simulink model "AdaptedGliderModel"  (R2019b)
settings: Solver=VariableStepAuto  StartTime=0.0  StopTime=10.0  RelTol=1e-3
undefined symbols (not defined in the file or in its folder): MDL
libraries: simulink x4, Driver_Glider_Library x2
settings Model: Creator=eduar  LastModifiedBy=eduar

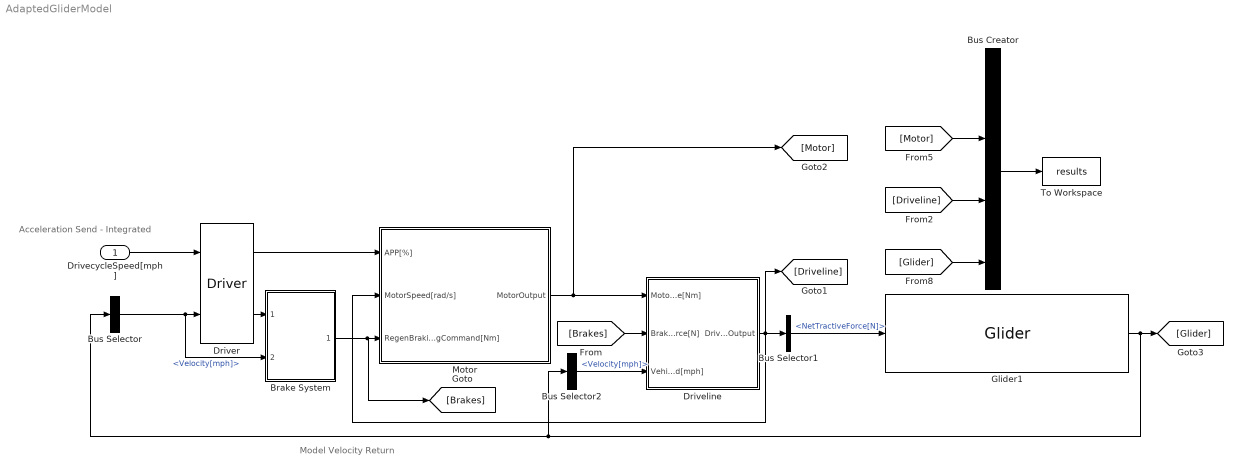
== system AdaptedGliderModel ==
  note: Model Velocity Return
  note: Acceleration Send - Integrated
  DrivecycleSpeed[mph] : Inport
  Brake System : Subsystem
      mask Display: image('brakes.jpg');
  Bus Creator : BusCreator  Inputs=4
  Bus Selector : BusSelector  OutputSignals=Velocity[mph]
  Bus Selector1 : BusSelector  OutputSignals=NetTractiveForce[N]
  Bus Selector2 : BusSelector  OutputSignals=Velocity[mph]
  Driveline : Subsystem
      mask Display: image('driveline.jpg');
  Driver : Driver_Glider_Library/Driver  SystemSampleTime=-1  Latency=0  AutoFrameSizeCalculation=off
  Glider1 : Driver_Glider_Library/Glider  SystemSampleTime=-1  Latency=0  AutoFrameSizeCalculation=off
      link override AerodynamicDrag[N]: Gain=0
      link override Force2Acceleration: Gain=1/388
      link override GradeForce[N]: Value=0
      link override RollingResistance[N]: Value=388*9.8*rollingResistCoeff
  Motor : Subsystem
      mask Display: image('motor.jpg');
  To Workspace : ToWorkspace  VariableName=results  SaveFormat=Timeseries  SampleTime=-1
  wires:
  Driver/1 -> Motor/1(APP[%])
  Bus Selector1/1 -> Glider1/1  "<NetTractiveForce[N]>"
  Bus Selector/1 -> Brake System/2(VehicleSpeed[mph]), Driver/2  "<Velocity[mph]>"
  Driver/2 -> Brake System/1(BPP[%])
  [Motor] -> Bus Creator/2
  DrivecycleSpeed[mph]/1 -> Driver/1
  Bus Creator/1 -> To Workspace/1
  Glider1/1 -> [Glider], Bus Selector/1, Bus Selector2/1
  [Driveline] -> Bus Creator/3
  Driveline/1(DrivelineOutput) -> Bus Selector1/1, Motor/2(MotorSpeed[rad/s]), [Driveline]
  Motor/1(MotorOutput) -> [Motor], Driveline/1(MotorTorque[Nm])
  [Glider] -> Bus Creator/4
  Brake System/1(BrakeOutput) -> [Brakes], Motor/3(RegenBrakingCommand[Nm])
  Bus Selector2/1 -> Driveline/3(VehicleSpeed[mph])  "<Velocity[mph]>"
  [Brakes] -> Driveline/2(BrakeForce[N])

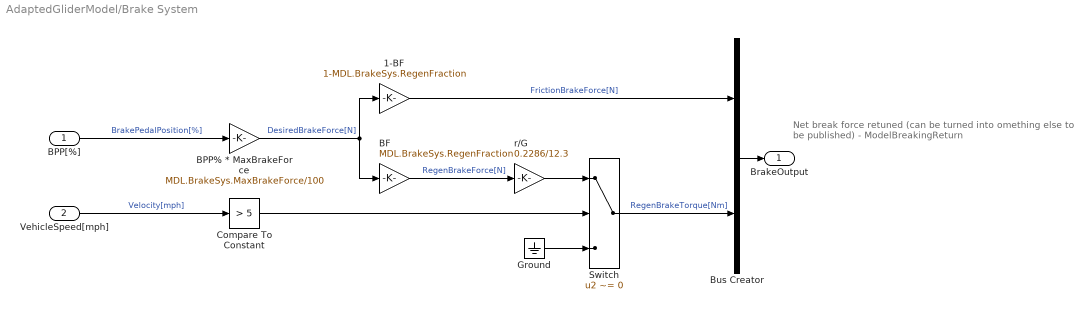
== system AdaptedGliderModel/Brake System ==
  note: Net break force retuned (can be turned into omething else
      | to be published) - ModelBreakingReturn
  BPP[%] : Inport
  VehicleSpeed[mph] : Inport  Port=2
  1-BF : Gain  Gain=1-MDL.BrakeSys.RegenFraction
  BF : Gain  Gain=MDL.BrakeSys.RegenFraction
  BPP% * MaxBrakeForce : Gain  Gain=MDL.BrakeSys.MaxBrakeForce/100
  Bus Creator : BusCreator  Inputs=2
  Compare To Constant : simulink/Logic and Bit Operations/Compare To Constant  relop=>  const=5  OutDataTypeStr=boolean
  Ground : Ground
  Switch : Switch  Criteria=u2 ~= 0
  r/G : Gain  Gain=0.2286/12.3
  BrakeOutput : Outport  VectorParamsAs1DForOutWhenUnconnected=off
  wires:
  Bus Creator/1 -> BrakeOutput/1
  BPP[%]/1 -> BPP% * MaxBrakeForce/1  "BrakePedalPosition[%]"
  BPP% * MaxBrakeForce/1 -> BF/1, 1-BF/1  "DesiredBrakeForce[N]"
  BF/1 -> r/G/1  "RegenBrakeForce[N]"
  1-BF/1 -> Bus Creator/1  "FrictionBrakeForce[N]"
  r/G/1 -> Switch/1
  VehicleSpeed[mph]/1 -> Compare To Constant/1  "Velocity[mph]"
  Ground/1 -> Switch/3
  Switch/1 -> Bus Creator/2  "RegenBrakeTorque[Nm]"
  Compare To Constant/1 -> Switch/2

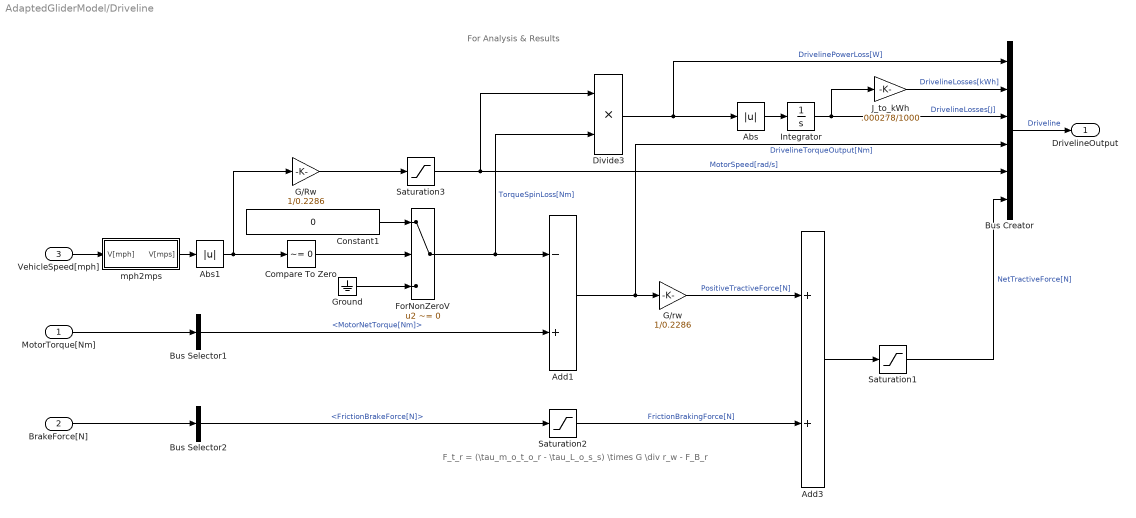
== system AdaptedGliderModel/Driveline ==
  note: For Analysis & Results
  note: F_t_r = (\tau_m_o_t_o_r - \tau_L_o_s_s) \times G \div r_w - F_B_r
  MotorTorque[Nm] : Inport
  BrakeForce[N] : Inport  Port=2
  VehicleSpeed[mph] : Inport  Port=3
  Abs : Abs  ZeroCross=off
  Abs1 : Abs  ZeroCross=off
  Add1 : Sum  Inputs=-+
  Add3 : Sum
  Bus Creator : BusCreator  Inputs=6
  Bus Selector1 : BusSelector  OutputSignals=MotorNetTorque[Nm]
  Bus Selector2 : BusSelector  OutputSignals=FrictionBrakeForce[N]
  Compare To Zero : simulink/Logic and Bit Operations/Compare To Zero  relop=~=  OutDataTypeStr=boolean
  Constant1 : Constant  Value=0
  Divide3 : Product  Inputs=**
  ForNonZeroV : Switch  Criteria=u2 ~= 0  ZeroCross=off
  G/Rw : Gain  Gain=1/0.2286
  G/rw : Gain  Gain=1/0.2286
  Ground : Ground
  Integrator : Integrator  ZeroCross=off
  J_to_kWh : Gain  Gain=.000278/1000
  Saturation1 : Saturate  UpperLimit=5000  LowerLimit=-10000  ZeroCross=off
  Saturation2 : Saturate  UpperLimit=0  LowerLimit=-10000  ZeroCross=off
  Saturation3 : Saturate  UpperLimit=inf  LowerLimit=0.00001  ZeroCross=off
  mph2mps : Subsystem
  DrivelineOutput : Outport  VectorParamsAs1DForOutWhenUnconnected=off
  wires:
  G/rw/1 -> Add3/1  "PositiveTractiveForce[N]"
  Add3/1 -> Saturation1/1
  Abs/1 -> Integrator/1
  BrakeForce[N]/1 -> Bus Selector2/1
  Saturation2/1 -> Add3/2  "FrictionBrakingForce[N]"
  MotorTorque[Nm]/1 -> Bus Selector1/1
  G/Rw/1 -> Saturation3/1
  VehicleSpeed[mph]/1 -> mph2mps/1(V[mph])
  ForNonZeroV/1 -> Divide3/2, Add1/1  "TorqueSpinLoss[Nm]"
  Add1/1 -> Bus Creator/4, G/rw/1  "DrivelineTorqueOutput[Nm]"
  Saturation3/1 -> Divide3/1, Bus Creator/5  "MotorSpeed[rad/s]"
  Divide3/1 -> Bus Creator/1, Abs/1  "DrivelinePowerLoss[W]"
  Saturation1/1 -> Bus Creator/6  "NetTractiveForce[N]"
  Abs1/1 -> Compare To Zero/1, G/Rw/1
  Bus Selector2/1 -> Saturation2/1  "<FrictionBrakeForce[N]>"
  J_to_kWh/1 -> Bus Creator/2  "DrivelineLosses[kWh]"
  Ground/1 -> ForNonZeroV/3
  Constant1/1 -> ForNonZeroV/1
  Bus Creator/1 -> DrivelineOutput/1  "Driveline"
  Integrator/1 -> J_to_kWh/1, Bus Creator/3  "DrivelineLosses[J]"
  Bus Selector1/1 -> Add1/2  "<MotorNetTorque[Nm]>"
  Compare To Zero/1 -> ForNonZeroV/2
  mph2mps/1(V[mps]) -> Abs1/1

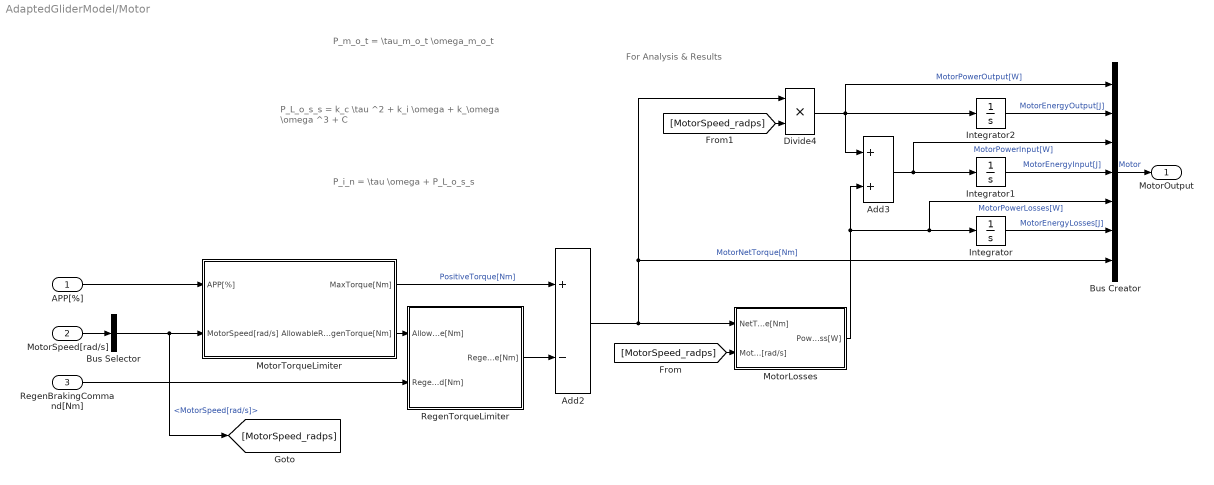
== system AdaptedGliderModel/Motor ==
  note: P_i_n = \tau \omega + P_L_o_s_s
  note: For Analysis & Results
  note: P_L_o_s_s = k_c \tau ^2 + k_i \omega + k_\omega \omega ^3 + C
  note: P_m_o_t = \tau_m_o_t \omega_m_o_t
  APP[%] : Inport
  MotorSpeed[rad/s] : Inport  Port=2
  RegenBrakingCommand[Nm] : Inport  Port=3
  Add2 : Sum  Inputs=+-
  Add3 : Sum
  Bus Creator : BusCreator  Inputs=7
  Bus Selector : BusSelector  OutputSignals=MotorSpeed[rad/s]
  Divide4 : Product  Inputs=**
  Integrator : Integrator  ZeroCross=off
  Integrator1 : Integrator  ZeroCross=off
  Integrator2 : Integrator  ZeroCross=off
  MotorLosses : Subsystem
  MotorTorqueLimiter : Subsystem
  RegenTorqueLimiter : Subsystem
  MotorOutput : Outport  VectorParamsAs1DForOutWhenUnconnected=off
  wires:
  Add3/1 -> Bus Creator/3, Integrator1/1  "MotorPowerInput[W]"
  Divide4/1 -> Bus Creator/1, Add3/1, Integrator2/1  "MotorPowerOutput[W]"
  [MotorSpeed_radps] -> Divide4/2
  Integrator1/1 -> Bus Creator/4  "MotorEnergyInput[J]"
  Integrator2/1 -> Bus Creator/2  "MotorEnergyOutput[J]"
  Add2/1 -> MotorLosses/1(NetTorque[Nm]), Divide4/1, Bus Creator/7  "MotorNetTorque[Nm]"
  MotorTorqueLimiter/1(MaxTorque[Nm]) -> Add2/1  "PositiveTorque[Nm]"
  APP[%]/1 -> MotorTorqueLimiter/1(APP[%])
  MotorLosses/1(PowerLoss[W]) -> Bus Creator/5, Integrator/1, Add3/2  "MotorPowerLosses[W]"
  RegenBrakingCommand[Nm]/1 -> RegenTorqueLimiter/2(RegenBrakeCommand[Nm])
  MotorTorqueLimiter/2(AllowableRegenTorque[Nm]) -> RegenTorqueLimiter/1(AllowableRegenTorque[Nm])
  RegenTorqueLimiter/1(RegenTorque[Nm]) -> Add2/2
  [MotorSpeed_radps] -> MotorLosses/2(MotorSpeed[rad/s])
  Bus Creator/1 -> MotorOutput/1  "Motor"
  Integrator/1 -> Bus Creator/6  "MotorEnergyLosses[J]"
  MotorSpeed[rad/s]/1 -> Bus Selector/1
  Bus Selector/1 -> MotorTorqueLimiter/2(MotorSpeed[rad/s]), [MotorSpeed_radps]  "<MotorSpeed[rad/s]>"

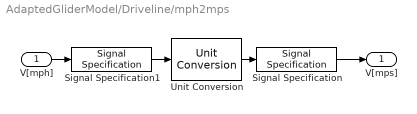
== system AdaptedGliderModel/Driveline/mph2mps ==
  V[mph] : Inport
  Signal Specification : SignalSpecification  Unit=m/s
  Signal Specification1 : SignalSpecification  Unit=mile/hr
  Unit Conversion : UnitConversion
  V[mps] : Outport  VectorParamsAs1DForOutWhenUnconnected=off
  wires:
  V[mph]/1 -> Signal Specification1/1
  Unit Conversion/1 -> Signal Specification/1
  Signal Specification1/1 -> Unit Conversion/1
  Signal Specification/1 -> V[mps]/1

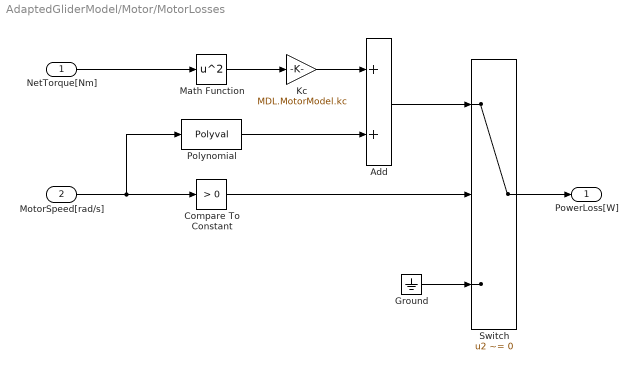
== system AdaptedGliderModel/Motor/MotorLosses ==
  NetTorque[Nm] : Inport
  MotorSpeed[rad/s] : Inport  Port=2
  Add : Sum
  Compare To Constant : simulink/Logic and Bit Operations/Compare To Constant  relop=>  const=0  OutDataTypeStr=boolean
  Ground : Ground
  Kc : Gain  Gain=MDL.MotorModel.kc
  Math Function : Math  Operator=square  SaturateOnIntegerOverflow=on
  Polynomial : Polyval  Coefs=[MDL.MotorModel.kw , 0 ,MDL.MotorModel.ki, MDL.MotorModel.C]
  Switch : Switch  Criteria=u2 ~= 0  ZeroCross=off
  PowerLoss[W] : Outport  VectorParamsAs1DForOutWhenUnconnected=off
  wires:
  NetTorque[Nm]/1 -> Math Function/1
  Math Function/1 -> Kc/1
  Kc/1 -> Add/1
  MotorSpeed[rad/s]/1 -> Polynomial/1, Compare To Constant/1
  Ground/1 -> Switch/3
  Switch/1 -> PowerLoss[W]/1
  Polynomial/1 -> Add/2
  Add/1 -> Switch/1
  Compare To Constant/1 -> Switch/2

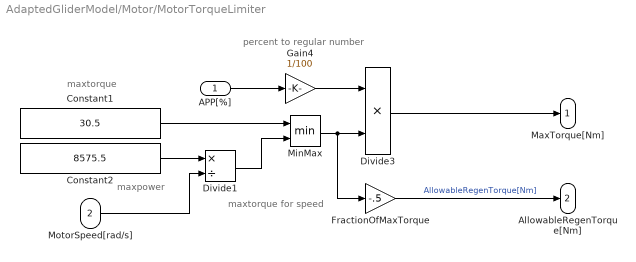
== system AdaptedGliderModel/Motor/MotorTorqueLimiter ==
  note: percent to regular number
  note: maxtorque for speed
  note: maxtorque
  note: maxpower
  APP[%] : Inport
  MotorSpeed[rad/s] : Inport  Port=2
  Constant1 : Constant  Value=30.5
  Constant2 : Constant  Value=8575.5
  Divide1 : Product  Inputs=*/
  Divide3 : Product  Inputs=**
  FractionOfMaxTorque : Gain  Gain=-.5
  Gain4 : Gain  Gain=1/100
  MinMax : MinMax  Inputs=2
  MaxTorque[Nm] : Outport  VectorParamsAs1DForOutWhenUnconnected=off
  AllowableRegenTorque[Nm] : Outport  Port=2  VectorParamsAs1DForOutWhenUnconnected=off
  wires:
  Constant1/1 -> MinMax/1
  MinMax/1 -> FractionOfMaxTorque/1, Divide3/2
  Gain4/1 -> Divide3/1
  APP[%]/1 -> Gain4/1
  Divide3/1 -> MaxTorque[Nm]/1
  Constant2/1 -> Divide1/1
  Divide1/1 -> MinMax/2
  MotorSpeed[rad/s]/1 -> Divide1/2
  FractionOfMaxTorque/1 -> AllowableRegenTorque[Nm]/1  "AllowableRegenTorque[Nm]"

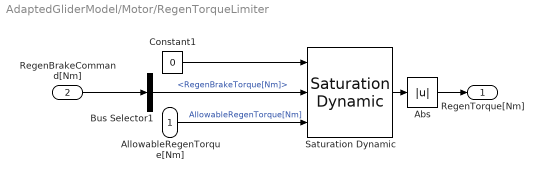
== system AdaptedGliderModel/Motor/RegenTorqueLimiter ==
  AllowableRegenTorque[Nm] : Inport
  RegenBrakeCommand[Nm] : Inport  Port=2
  Abs : Abs
  Bus Selector1 : BusSelector  OutputSignals=RegenBrakeTorque[Nm]
  Constant1 : Constant  Value=0
  Saturation Dynamic : simulink/Discontinuities/Saturation Dynamic  OutMin=[]  OutMax=[]  OutDataTypeStr=Inherit: Same as second input  OutDataType=fixdt(1, 16)  OutScaling=2^-10  DoSatur=off
  RegenTorque[Nm] : Outport  VectorParamsAs1DForOutWhenUnconnected=off
  wires:
  AllowableRegenTorque[Nm]/1 -> Saturation Dynamic/3  "AllowableRegenTorque[Nm]"
  Constant1/1 -> Saturation Dynamic/1
  Bus Selector1/1 -> Saturation Dynamic/2  "<RegenBrakeTorque[Nm]>"
  RegenBrakeCommand[Nm]/1 -> Bus Selector1/1
  Saturation Dynamic/1 -> Abs/1
  Abs/1 -> RegenTorque[Nm]/1
